simulink model "LQR1_Sim"  (R2020a)
settings: Solver=FixedStepAuto  StartTime=0.0  StopTime=100  FixedStep=1e-2  RelTol=1e-3
settings Model: Creator=niran  LastModifiedBy=niranjan.bhujel

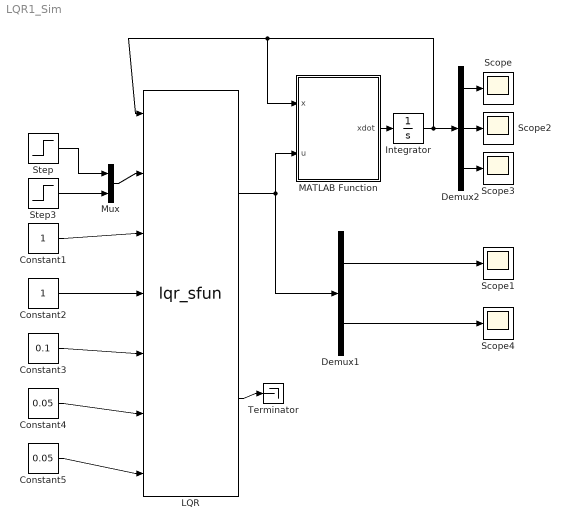
== system LQR1_Sim ==
  Constant1 : Constant
  Constant2 : Constant
  Constant3 : Constant  Value=0.1
  Constant4 : Constant  Value=0.05
  Constant5 : Constant  Value=0.05
  Demux1 : Demux  Outputs=2
  Demux2 : Demux  Outputs=3
  Integrator : Integrator
  LQR : S-Function  InitFcn=try, set_param(gcb,'FunctionName','lqr_sfun'), end  FunctionName=lqr_sfun  SFunctionModules=lqr_sfun_wrapper lqr_code lqr_code_Call  SFunctionDeploymentMode=off  EnableBusSupport=off  mask(S-Function Builder){}
      mask help: Simulink:masks:SFunctionBuilder_MD
      mask init:
      | val = [[.9  0.75 0.75 1 1 .9 .9 1]',[1 1 0.75 0.75 .9 .9 1 .9]'];try , sys = get_param(gcb,'SfunBuilderFcnName');if isempty(sys), sys = get_param(gcb,'FunctionName'); end,catch, sys = get_param(gcb,'FunctionName'); end
      settings: CopyFcn=set_param(gcbh,'LinkStatus','none')  PreSaveFcn=try, set_param(gcb,'FunctionName','lqr_sfun'), end  OpenFcn=sfunctionwizard(gcbh)
      mask Display: plot(val(:,1),val(:,2)),disp(sys), port_label('input',1,'x'), port_label('input',2,'ref'), port_label('input',3,'Q11'), port_label('input',4,'Q22'), port_label('input',5,'Q33'), port_label('input',6,'R11'), port_label('input',7,'R22'), port_label('output',1,'u'), port_label('output',2,'K')
  MATLAB Function : MATLAB Function  TreatAsAtomicUnit=on
  Mux : Mux  Inputs=2
  Scope{,1..4} (5 alike) : Scope
  Step : Step  Time=50  Before=0.5  SampleTime=0
  Step3 : Step  Time=75  Before=25  After=35  SampleTime=0
  Terminator : Terminator
  wires:
  Constant2/1 -> LQR/4
  Constant1/1 -> LQR/3
  LQR/1 -> Demux1/1, MATLAB Function/2(u)
  Mux/1 -> LQR/2
  Step/1 -> Mux/1
  Step3/1 -> Mux/2
  Constant3/1 -> LQR/5
  Constant4/1 -> LQR/6
  Constant5/1 -> LQR/7
  Demux1/1 -> Scope1/1
  Demux1/2 -> Scope4/1
  LQR/2 -> Terminator/1
  MATLAB Function/1(xdot) -> Integrator/1
  Integrator/1 -> MATLAB Function/1(x), LQR/1, Demux2/1
  Demux2/1 -> Scope/1
  Demux2/2 -> Scope2/1
  Demux2/3 -> Scope3/1

== matlab function LQR1_Sim/MATLAB Function ==
  data: x input; u input; xdot output
function xdot = fcn(x, u)
    xdot = zeros(3, 1);
    A = [-0.4, 0.1, -2.0;
        0, -0.3, 4.0;
        1.0, 0.0, 0.0];
    B = [1, 1;
        0, 1;
        1, 0];
    
    xdot = A * x + B * u;
end
